simulink model "Fahrzeugmodell_Sprungantwort"  (Simulink 8.3)
settings: Solver=ode45  StartTime=0.0  StopTime=10.0  MaxStep=1e-3  RelTol=1e-3
values from neighbouring files (symbols this model uses):
  c = 55270    [Fahrzeugmodell_Parameter.m]
  d = 3079    [Fahrzeugmodell_Parameter.m]
  l0 = 0.5    [Fahrzeugmodell_Parameter.m]
  mA = 1400    [Fahrzeugmodell_Parameter.m]
  T1 = 5e-3    (= 0.005)    [Fahrzeugmodell_Parameter.m]
  y0 = l0 - mA*g/c    (= 0.251510765334)    [Fahrzeugmodell_Parameter.m]
libraries: simulink x1
settings Model: Creator=Glöckler  LastModifiedBy=Glöckler
settings OptimizationCC: ExpressionDepthLimit=2147483647
settings DebuggingCC: FcnCallInpInsideContextMsg=UseLocalSettings

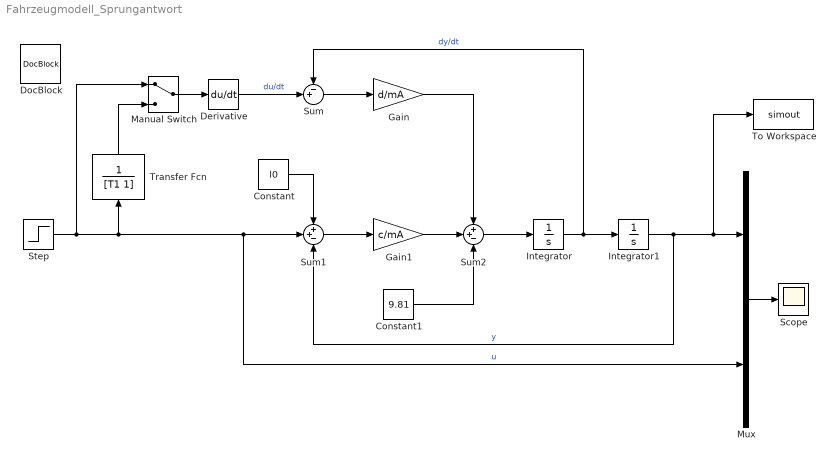
== system Fahrzeugmodell_Sprungantwort ==
  Constant : Constant  Value=l0
  Constant1 : Constant  Value=9.81
  Derivative : Derivative
  DocBlock : simulink/Model-Wide Utilities/DocBlock  DocumentType=Text
      content=|
      | Simulink-Modell des Fahrzeugmodells,
      |
      | Das Fahrzeug wird hier durch einen Sprung nach 4s angeregt;
      | Eingangsgröße x und Ausgangsgröße y werden im Scope angezeigt.
      |
      | Anfangswert y(0) = y0 steht im Block Integrator1
      |
      | Der Block Transfer Fcn beinhaltet ein PT1-Gleid als Tiefpassfilter.
      |
      | Der Block Manual Switch dient zum Ein/Ausschalten des Tiefpassfilters.
  Gain : Gain  Gain=d/mA
  Gain1 : Gain  Gain=c/mA
  Integrator : Integrator
  Integrator1 : Integrator  InitialCondition=y0
  Manual Switch : ManualSwitch
  Mux : Mux  Inputs=2
  Scope : Scope
      settings: TimeRange=10  YMin=0  YMax=0.35
  Step : Step  Time=4  After=0.05  SampleTime=0
  Sum : Sum  Inputs=-+|
  Sum1 : Sum  Inputs=++-
  Sum2 : Sum  Inputs=++-
  To Workspace : ToWorkspace  VariableName=simout  SaveFormat=Structure With Time  SampleTime=-1
  Transfer Fcn : TransferFcn  Denominator=[T1 1]
  wires:
  Derivative/1 -> Sum/2  "du/dt"
  Step/1 -> Manual Switch/1, Mux/2, Sum1/2, Transfer Fcn/1  "u"
  Constant/1 -> Sum1/1
  Sum/1 -> Gain/1
  Sum1/1 -> Gain1/1
  Gain1/1 -> Sum2/2
  Gain/1 -> Sum2/1
  Constant1/1 -> Sum2/3
  Sum2/1 -> Integrator/1
  Integrator/1 -> Integrator1/1, Sum/1  "dy/dt"
  Integrator1/1 -> Sum1/3, Mux/1, To Workspace/1  "y"
  Mux/1 -> Scope/1
  Manual Switch/1 -> Derivative/1
  Transfer Fcn/1 -> Manual Switch/2
